simulink model "failure_detection"  (R2021a)
settings: Solver=VariableStepAuto  StartTime=0.0  StopTime=10.0  RelTol=1e-3
libraries: simulink x2
settings Model: Creator=Beshary  LastModifiedBy=Beshary
settings DataIOCC: InspectSignalLogs=on

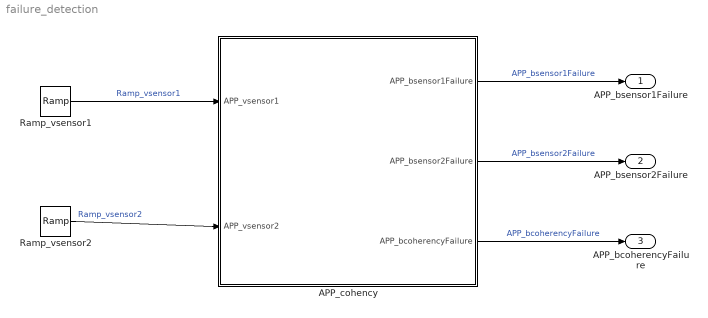
== system failure_detection ==
  APP_cohency : Subsystem
  Ramp_vsensor1 : simulink/Sources/Ramp  slope=0.4  start=0  InitialOutput=0.5
  Ramp_vsensor2 : simulink/Sources/Ramp  slope=-0.4  start=0  InitialOutput=5
  APP_bsensor1Failure : Outport
  APP_bsensor2Failure : Outport  Port=2
  APP_bcoherencyFailure : Outport  Port=3
  wires:
  Ramp_vsensor1/1 -> APP_cohency/1(APP_vsensor1)  "Ramp_vsensor1"
  Ramp_vsensor2/1 -> APP_cohency/2(APP_vsensor2)  "Ramp_vsensor2"
  APP_cohency/1(APP_bsensor1Failure) -> APP_bsensor1Failure/1  "APP_bsensor1Failure"
  APP_cohency/2(APP_bsensor2Failure) -> APP_bsensor2Failure/1  "APP_bsensor2Failure"
  APP_cohency/3(APP_bcoherencyFailure) -> APP_bcoherencyFailure/1  "APP_bcoherencyFailure"

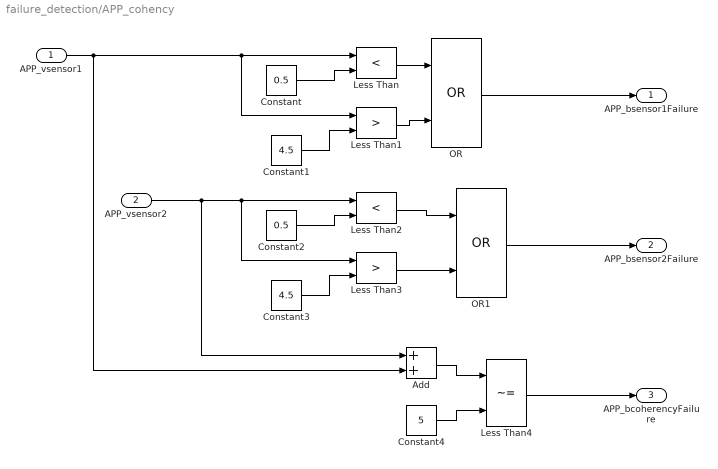
== system failure_detection/APP_cohency ==
  APP_vsensor1 : Inport
  APP_vsensor2 : Inport  Port=2
  Add : Sum
  Constant : Constant  Value=0.5
  Constant1 : Constant  Value=4.5
  Constant2 : Constant  Value=0.5
  Constant3 : Constant  Value=4.5
  Constant4 : Constant  Value=5
  Less Than : RelationalOperator  Operator=<  OutDataTypeStr=boolean  RndMeth=Simplest
  Less Than1 : RelationalOperator  Operator=>  OutDataTypeStr=boolean  RndMeth=Simplest
  Less Than2 : RelationalOperator  Operator=<  OutDataTypeStr=boolean  RndMeth=Simplest
  Less Than3 : RelationalOperator  Operator=>  OutDataTypeStr=boolean  RndMeth=Simplest
  Less Than4 : RelationalOperator  Operator=~=  OutDataTypeStr=boolean  RndMeth=Simplest
  OR : Logic  Operator=OR  AllPortsSameDT=off  OutDataTypeStr=boolean
  OR1 : Logic  Operator=OR  AllPortsSameDT=off  OutDataTypeStr=boolean
  APP_bsensor1Failure : Outport
  APP_bsensor2Failure : Outport  Port=2
  APP_bcoherencyFailure : Outport  Port=3
  wires:
  APP_vsensor1/1 -> Add/2, Less Than1/1, Less Than/1
  Constant/1 -> Less Than/2
  Less Than/1 -> OR/1
  Constant1/1 -> Less Than1/2
  Less Than1/1 -> OR/2
  OR/1 -> APP_bsensor1Failure/1
  Constant3/1 -> Less Than3/2
  Constant2/1 -> Less Than2/2
  APP_vsensor2/1 -> Add/1, Less Than3/1, Less Than2/1
  Less Than2/1 -> OR1/1
  Less Than3/1 -> OR1/2
  OR1/1 -> APP_bsensor2Failure/1
  Add/1 -> Less Than4/1
  Constant4/1 -> Less Than4/2
  Less Than4/1 -> APP_bcoherencyFailure/1
